simulink model "MPC_LQR"  (R2025b)
settings: Solver=ode4  StartTime=0.0  StopTime=10  FixedStep=0.001  RelTol=1e-3
InitFcn:
  | run("init.m")
settings Model: Creator=aldor  LastModifiedBy=Acer

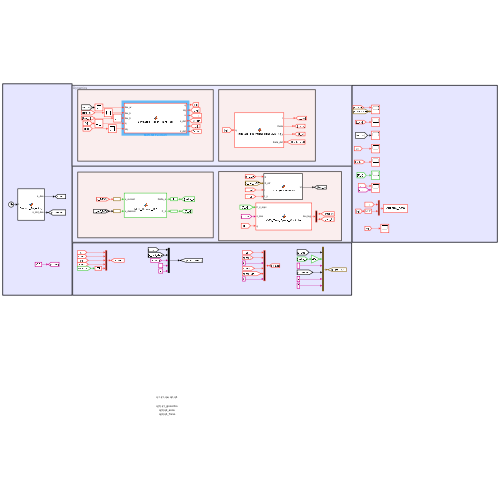
[thumbnail: Simulink's stored preview of the top-level diagram]
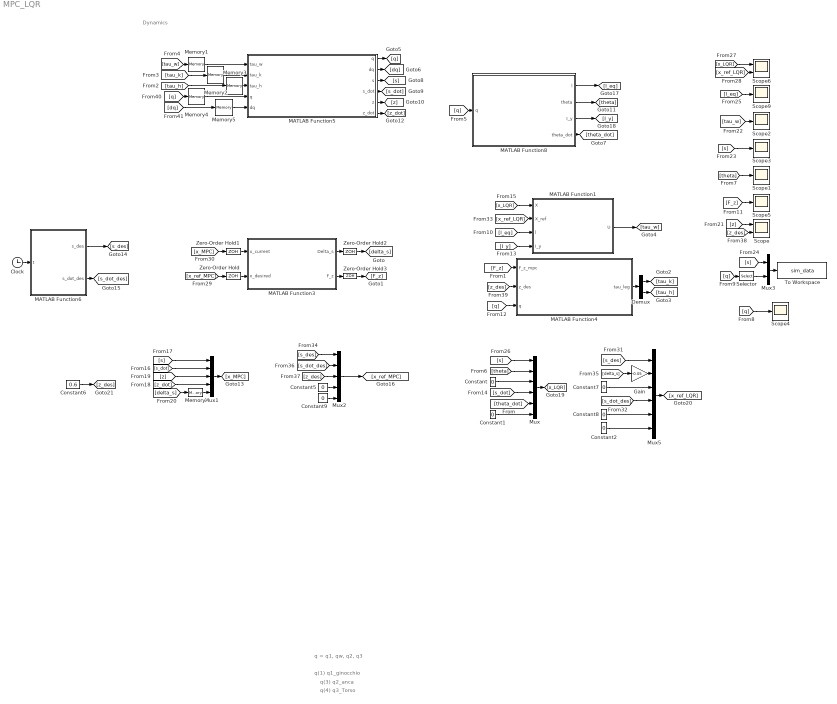
== system MPC_LQR ==
  note: Dynamics
  note: q(3) q2_anca
  note: q(1) q1_ginocchio
  note: q = q1, qw, q2, q3
  note: q(4) q3_Torso
  Clock : Clock
  Constant{,1..2,5,7..9} (7 alike) : Constant  Value=0
  Constant6 : Constant  Value=0.6
  Demux : Demux  Outputs=2
  Gain : Gain  Gain=-0.05
  MATLAB Function1 : MATLAB Function  TreatAsAtomicUnit=on
  MATLAB Function3 : MATLAB Function  TreatAsAtomicUnit=on
  MATLAB Function4 : MATLAB Function  TreatAsAtomicUnit=on
  MATLAB Function5 : MATLAB Function  TreatAsAtomicUnit=on
  MATLAB Function6 : MATLAB Function  TreatAsAtomicUnit=on
  MATLAB Function8 : MATLAB Function  TreatAsAtomicUnit=on
  Memory{,1..5} (6 alike) : Memory
  Mux : Mux  Inputs=6
  Mux1 : Mux  Inputs=5
  Mux2 : Mux  Inputs=5
  Mux3 : Mux  Inputs=[1 3]
  Mux5 : Mux  Inputs=6
  Scope : Scope  NumInputPorts=2
      settings: ActiveDisplayYMinimum=0.1067548531401226  ActiveDisplayYMaximum=0.98813834965109748
  Scope{1..5,9} (6 alike) : Scope
      Scope1 settings: ActiveDisplayYMinimum=-0.026598662061855207  ActiveDisplayYMaximum=0.032394796278817736
      Scope2 settings: ActiveDisplayYMinimum=-998.36065850881471  ActiveDisplayYMaximum=2321.7471304243586  DataLoggingVariableName=ScopeData2
      Scope3 settings: ActiveDisplayYMinimum=-0.15390799680390416  ActiveDisplayYMaximum=1.2448530557444439  DataLoggingVariableName=ScopeData3
      Scope4 settings: ActiveDisplayYMinimum=-1  ActiveDisplayYMaximum=1  DataLoggingVariableName=ScopeData4
      Scope5 settings: ActiveDisplayYMinimum=-792.61159771990333  ActiveDisplayYMaximum=837.79442871292474  DataLoggingVariableName=ScopeData5
      Scope9 settings: ActiveDisplayYMinimum=0.26491553159842146  ActiveDisplayYMaximum=1.1125448908081954  DataLoggingVariableName=ScopeData9
  Scope6 : Scope  NumInputPorts=2
      settings: ActiveDisplayYMinimum=-1  ActiveDisplayYMaximum=1  DataLoggingVariableName=ScopeData6
  Selector : Selector  InputPortWidth=4  IndexOptions=Index vector (dialog)  Indices=[1 3 4]  OutputSizes=1
  To Workspace : ToWorkspace  VariableName=sim_data  SampleTime=-1
  Zero-Order Hold{,1..3} (4 alike) : ZeroOrderHold  SampleTime=1e-2
  wires:
  MATLAB Function4/1(tau_leg) -> Demux/1
  Demux/1 -> [tau_k]
  Demux/2 -> [tau_h]
  MATLAB Function5/1(q) -> [q]
  MATLAB Function5/2(dq) -> [dq]
  MATLAB Function5/5(z) -> [z]
  MATLAB Function5/3(s) -> [s]
  MATLAB Function5/4(s_dot) -> [s_dot]
  [s] -> Mux/1
  Constant/1 -> Mux/3
  [s_dot] -> Mux/4
  Mux/1 -> [x_LQR]
  [x_LQR] -> MATLAB Function1/1(X)
  [x_ref_LQR] -> MATLAB Function1/2(X_ref)
  [s_dot] -> Mux1/2
  [s] -> Mux1/1
  [z] -> Mux1/3
  [z_dot] -> Mux1/4
  [delta_s] -> Memory/1
  Memory/1 -> Mux1/5
  Constant5/1 -> Mux2/4
  Constant9/1 -> Mux2/5
  [tau_w] -> Memory1/1
  Memory1/1 -> MATLAB Function5/1(tau_w)
  Memory2/1 -> MATLAB Function5/2(tau_k)
  [tau_k] -> Memory2/1
  [tau_h] -> Memory3/1
  Memory3/1 -> MATLAB Function5/3(tau_h)
  [z] -> Scope/1
  [z_des] -> Scope/2
  [tau_w] -> Scope2/1
  [s] -> Scope3/1
  Mux3/1 -> To Workspace/1
  [s] -> Mux3/1
  Clock/1 -> MATLAB Function6/1(t)
  MATLAB Function6/1(s_des) -> [s_des]
  [z_des] -> Mux2/3
  [s_des] -> Mux5/1
  [s_dot_des] -> Mux5/4
  Mux5/1 -> [x_ref_LQR]
  [F_z] -> Scope5/1
  [F_z] -> MATLAB Function4/1(F_z_mpc)
  [delta_s] -> Gain/1
  Gain/1 -> Mux5/2
  Mux2/1 -> [x_ref_MPC]
  Zero-Order Hold/1 -> MATLAB Function3/2(x_desired)
  Zero-Order Hold1/1 -> MATLAB Function3/1(x_current)
  Mux1/1 -> [x_MPC]
  Zero-Order Hold2/1 -> [delta_s]
  MATLAB Function3/1(Delta_s) -> Zero-Order Hold2/1
  MATLAB Function3/2(F_z) -> Zero-Order Hold3/1
  Zero-Order Hold3/1 -> [F_z]
  MATLAB Function5/6(z_dot) -> [z_dot]
  [q] -> MATLAB Function4/3(q)
  [q] -> MATLAB Function8/1(q)
  MATLAB Function8/4(theta_dot) -> [theta_dot]
  [theta_dot] -> Mux/5
  Constant1/1 -> Mux/6
  MATLAB Function8/2(theta) -> [theta]
  [theta] -> Mux/2
  [theta] -> Scope1/1
  [q] -> Scope4/1
  [q] -> Selector/1
  Selector/1 -> Mux3/2
  MATLAB Function8/1(l) -> [l_eq]
  [l_eq] -> MATLAB Function1/3(l)
  [l_eq] -> Scope9/1
  MATLAB Function8/3(I_y) -> [I_y]
  [I_y] -> MATLAB Function1/4(I_y)
  [x_LQR] -> Scope6/1
  [x_ref_LQR] -> Scope6/2
  Constant2/1 -> Mux5/6
  Constant8/1 -> Mux5/5
  Constant7/1 -> Mux5/3
  [x_ref_MPC] -> Zero-Order Hold/1
  [x_MPC] -> Zero-Order Hold1/1
  MATLAB Function6/2(s_dot_des) -> [s_dot_des]
  [s_dot_des] -> Mux2/2
  [s_des] -> Mux2/1
  Constant6/1 -> [z_des]
  [z_des] -> MATLAB Function4/2(z_des)
  [q] -> Memory4/1
  [dq] -> Memory5/1
  MATLAB Function1/1(U) -> [tau_w]
  Memory4/1 -> MATLAB Function5/4("q ")
  Memory5/1 -> MATLAB Function5/5("dq ")

== matlab function MPC_LQR/MATLAB Function1 ==
  data: X input; U output; X_ref input; l input; I_y input
function U = TV_LQR_Controller(X, X_ref, l, I_y)
    % X: Stato attuale [s; theta; phi; s_dot; theta_dot; phi_dot] (6x1)
    % X_ref: Stato target desiderato [s_ref; theta_ref; phi_ref; 0; 0; 0] (6x1)
    % l: Lunghezza attuale del pendolo equivalente [m]
    % I_y: Inerzia attuale del corpo superiore [kg*m^2]
    
    % Per usare la funzione lqr() di MATLAB all'interno di Simulink, 
    % dobbiamo dichiararla come estrinseca.
    coder.extrinsic('lqr');
    if l < 0.1
        l = 0.1;
    end
    if I_y < 1e-3
        I_y = 1e-3;
    end
    % 1. Richiamo Parametri Fisici
    m_w = 3.5;       % Massa ruota
    I_w = 0.1;       % Inerzia ruota
    r   = 0.127;     % Raggio ruota
    d   = 0.63;      % Distanza ruote
    m_b = 73.0;      % Massa corpo superiore
    I_z = 3.3;       % Inerzia torso asse z
    g   = 9.81;      % Gravità
    
    % 2. Calcolo dei Coefficienti della Dinamica (Eq. 14)
    % Denominatore comune per a1, a2, b1, b2
    D = 2*I_w*(I_y + m_b*l^2) + (2*l^2*m_b*m_w + I_y*(m_b + 2*m_w)*r^2);
    
    a1 = -(g * l^2 * m_b^2 * r^2) / D;
    a2 =  (g * l * m_b * (2*I_w + (m_b + 2*m_w)*r^2)) / D;
    
    b1 =  (r * (I_y + l*m_b*(l + r))) / D;
    b2 = -(2*I_w + r*(l*m_b + (m_b + 2*m_w)*r)) / D;
    
    % Coefficiente disaccoppiato per lo steering (imbardata)
    b3 =  (d * r) / (2*I_z*r^2 + d^2*(I_w + m_w*r^2));
    
    % 3. Costruzione Matrici di Stato A(l) e Input B(l) (Eq. 12, Eq. 13)
    A = zeros(6, 6);
    A(1, 4) = 1; 
    A(2, 5) = 1; 
    A(3, 6) = 1;
    A(4, 2) = a1;
    A(5, 2) = a2;
    
    B = zeros(6, 2);
    B(4, 1) = b1;  B(4, 2) = b1;
    B(5, 1) = b2;  B(5, 2) = b2;
    B(6, 1) = b3;  B(6, 2) = -b3;
    
    % 4. Definizione Matrici di Peso Q e R (Tuning LQR)
    % Questi valori determinano l'aggressività del controllore. 
    % Possono essere trasformati in input del blocco per un tuning rapido.
    % 4. Definizione Matrici di Peso Q e R (Tuning Soft)
    % Pesi drasticamente ridotti per evitare instabilità con il ritardo discreto
% Aumenta il peso sugli angoli (q1, q2) per evitare che saturino
%X = [s, θ, φ, ṡ, θ̇, φ̇]
    Q = diag([50, 50, 100, 50, 10, 1]);
    R = diag([1, 1]) * 0.5;         % uso coppie piu abbasso piu accelera
    
    % 5. Risoluzione LQR e Calcolo Input
    % Inizializza K per la Code Generation di Simulink
    K = zeros(2, 6); 
    
    % Calcola la matrice dei guadagni ottimali K
    K = lqr(A, B, Q, R);
    
    % Errore di stato (tilde_X)
    X_tilde = X - X_ref;
    
    % Legge di controllo finale (Eq. 16): U = [tau_l; tau_r]
    U = -K * X_tilde; 
end

== matlab function MPC_LQR/MATLAB Function3 ==
  data: x_current input; Delta_s output; x_desired input; F_z output
function [Delta_s, F_z] = MPC_Custom_QP(x_current, x_desired)
    % quadprog non è supportato nativamente per la code generation C
    coder.extrinsic('quadprog');
    coder.extrinsic('optimoptions');

    %% 1. Parametri e Discretizzazione
    m_b = 73.0; 
    g = 9.81;    
    
    h = x_current(3); 
    if h < 0.1
        h = 0.6;
    end
    
    dt = 0.01; 
    N = 40;     
    
    A_c = zeros(5,5);
    A_c(1,2) = 1;
    A_c(3,4) = 1;
    A_c(2,5) = g / h; 
    
    B_c = zeros(5,2);
    B_c(4,2) = 1 / m_b;
    B_c(5,1) = 1;
    
    A_d = eye(5) + A_c * dt;
    B_d = B_c * dt;

    %% 2. Pesi della Funzione di Costo
    %x = [s, ṡ, z, ż, Δs]
    S = diag([1, 1, 500, 50, 1]);
    W = diag([1, 0.01]);

    %% 3. Condensazione (Srotolamento) 
    nx = 5; nu = 2;
    P_x = zeros(nx*N, nx);
    P_u = zeros(nx*N, nu*N);

    A_power = eye(nx);
    for i = 1:N
        A_power = A_power * A_d;
        P_x((i-1)*nx+1 : i*nx, :) = A_power;
        for j = 1:i
            P_u((i-1)*nx+1 : i*nx, (j-1)*nu+1 : j*nu) = (A_d^(i-j)) * B_d;
        end
    end

    S_bar = kron(eye(N), S);
    W_bar = kron(eye(N), W);

    H = 2 * (P_u' * S_bar * P_u + W_bar);
    H = (H + H') / 2; % Garantisce simmetria perfetta
    
    X_ref = repmat(x_desired, N, 1);
    f = 2 * P_u' * S_bar * (P_x * x_current - X_ref);

    %% 4. Vincoli Fisici
    F_min = -1500; % Permette di frenare!
    F_max = 1500;
    
    LB = zeros(nu*N, 1);
    UB = zeros(nu*N, 1);
    
    for i = 1:N
        LB((i-1)*nu+1) = -0.20;   % era -2.0

        UB((i-1)*nu+1) =  0.20;   % era  2.0
 
        
        LB((i-1)*nu+2) = F_min; 
        UB((i-1)*nu+2) = F_max;
    end

    %% 5. Risoluzione QP (CORRETTA)
    % Pre-allocazione per Simulink Coder
    U_opt_calc = zeros(nu*N, 1);
    fval = 0.0;
    exitflag = 0.0;
    
    % Algoritmo robusto di default
    options = optimoptions('quadprog', 'Display', 'off');
    
    % LA CORREZIONE: Aggiunto "fval" per non sballare "exitflag"!
    [U_opt_calc, fval, exitflag] = quadprog(H, f, [], [], [], [], LB, UB, [], options);

    if exitflag > 0
        U_opt = U_opt_calc;
    else
        % Se fallisce davvero, eroga 0 extra, ma il VMC ci terrà in piedi col peso base
        U_opt = zeros(nu*N, 1);
    end

    %% 6. Estrazione Input Ottimo
    Delta_s_dot_opt = U_opt(1);
    F_z = U_opt(2); % FINALMENTE SARA' DIVERSO DA ZERO!

    Delta_s = x_current(5) + Delta_s_dot_opt * dt;
end

== matlab function MPC_LQR/MATLAB Function4 ==
  settings: updateMethod=DISCRETE
  data: tau_leg output size=2; F_z_mpc input size=1; z_des input size=1; q input size=4
function tau_leg  = VMC_Task_Space_Controller(F_z_mpc, z_des, q)

% =========================================================================

% VMC CORRETTO - Ripartizione pulita delle competenze della GAMBA:

%   GINOCCHIO -> altezza z          (canale verticale)

%   ANCA      -> beccheggio torso q3 (stabilizzazione, anello prima mancante)

% Lo spostamento ORIZZONTALE del CoM NON e' piu' gestito qui: e' compito

% della ruota (TV-LQR). Cosi' sparisce il conflitto che destabilizzava l'MPC.

% =========================================================================

    % --- Parametri fisici ---

    l1 = 0.45; l2 = 0.45;

    dt    = 0.001;        % deve coincidere col passo fisso del solutore
 
    % --- Stima derivate via differenza finita (persistenti) ---


 
    % Cinematica utile

    q1_ginocchio=q(1);
    q2_anca=q(3);
    q3_torso=q(4);

        persistent q3_prev z_prev

    if isempty(q3_prev), q3_prev = q3_torso; end

    phi_shank = q1_ginocchio - q2_anca + q3_torso;

    phi_thigh = q3_torso - q2_anca;

    z_actual  = l1*cos(phi_shank) + l2*cos(phi_thigh);
 
    if isempty(z_prev), z_prev = z_actual; end
 
    dq3   = (q3_torso - q3_prev)/dt;   q3_prev = q3_torso;

    z_dot = (z_actual - z_prev)/dt;    z_prev  = z_actual;
 
    % --- CoM: solo per monitoraggio/uscite ---

    coder.extrinsic('calc_com_jacobian');

    J_SC = zeros(1,2); J_ZC = zeros(1,2); SC = 0.0; ZC = 0.0;

    [J_SC, J_ZC, SC, ZC] = calc_com_jacobian(q1_ginocchio, q2_anca, q3_torso);

    SC_out    = SC;

    J_hip_out = J_SC(2);
 
    % --- Compensazione di gravita' dalla dinamica VERA G(q) ---

    % (sostituisce il vecchio Jacobiano del ginocchio "clampato", instabile

    %  a gamba dritta). G non dipende da dq, quindi passo dq = 0.

    coder.extrinsic('calc_dynamics');

    q_full  = [q1_ginocchio; 0; q2_anca; q3_torso];   % ordine [q1;qw;q2;q3]

    M   = zeros(4,4); CdQ = zeros(4,1); G = zeros(4,1);

    [M, CdQ, G] = calc_dynamics(q_full, zeros(4,1));

    tau_k_grav = G(1);   % coppia statica ginocchio

    tau_h_grav = G(3);   % coppia statica anca
 
    % =====================================================================

    % (1) GINOCCHIO  ->  controllo di ALTEZZA

    % =====================================================================

    Kp_z = 4000; Kd_z = 300;               % PD altezza (DA TARARE)

    Jz_knee = -l1*sin(phi_shank);          % dz/dq1

    if abs(Jz_knee) < 0.05                  % vicino a gamba dritta: autorita' ~0

        Jz_knee = 0.05*sign(Jz_knee + 1e-9);

    end

    F_z_cmd = Kp_z*(z_des - z_actual) - Kd_z*z_dot + F_z_mpc;  % forza vert. extra

    tau_k   = tau_k_grav + Jz_knee * F_z_cmd;
 
    % =====================================================================

    % (2) ANCA  ->  stabilizza il BECCHEGGIO del torso  q3 -> 0

    % =====================================================================

    Kp_t = 800; Kd_t = 80;                 % PD torso (DA TARARE)

    % SEGNO: parti con -(Kp*q3 + Kd*dq3). Se in simulazione il torso DIVERGE

    %        invece di raddrizzarsi, INVERTI il segno del termine PD.

    tau_h = tau_h_grav - (Kp_t*q3_torso + Kd_t*dq3);
 
    tau_leg = [tau_k; tau_h];

end

== matlab function MPC_LQR/MATLAB Function5 ==
  data: tau_w input size=2; q output; tau_k input size=1; tau_h input size=1; dq output; s output size=1; s_dot output size=1; z output size=1; z_dot output size=1; q input size=4; dq input size=4
function [q, dq, s, s_dot, z, z_dot] = Simulated_Robot_Plant_Full(tau_w, tau_k, tau_h, q, dq)

    persistent q_static dq_static
    if isempty(q_static)
        q_static  = [0; 0; 0; 0];
        dq_static = [0; 0; 0; 0];
    end

    dt = 0.001;
    limite_gamba = 300;limite_ruota = 50; 
    tau_w_scalar = max(min(tau_w(1)+tau_w(2), limite_ruota), -limite_ruota);
    tau_k_lim    = max(min(tau_k, limite_gamba), -limite_gamba);
    tau_h_lim    = max(min(tau_h, limite_gamba), -limite_gamba);

    tau_vec = [tau_k_lim; tau_w_scalar; tau_h_lim; 0];

    ddq = whole_robot_2D(q, dq, tau_vec);
    dq_static  = dq_static + ddq * dt;
    q_static   = q_static  + dq_static * dt;

    q1_ginocchio = q_static(1);
    q2_anca      = q_static(3);
    q3_torso     = q_static(4); 

    Rw = 0.127;
    s = Rw * q_static(2);
    s_dot    = Rw * dq_static(2);

    l1 = 0.45; l2 = 0.45;
    phi_shank = q1_ginocchio - q2_anca + q3_torso;
    phi_thigh = q3_torso - q2_anca;
    z = l1*cos(phi_shank) + l2*cos(phi_thigh);

    persistent z_prev
    if isempty(z_prev), z_prev = z; end
    z_dot = (z - z_prev)/dt;
    z_prev = z;

    q=q_static;
    dq=dq_static;
end

== matlab function MPC_LQR/MATLAB Function6 ==
  data: t input; s_des output; s_dot_des output
function [s_des, s_dot_des] = Smooth_Trajectory(t)
    % PRE-ALLOCAZIONE PER IL CODER
    s_des = 0.0;
    s_dot_des = 0.0;
    
    % PARAMETRI DELLA TRAIETTORIA
    t_start = 0.0;       % Il robot inizia a muoversi a 2 secondi
    t_end = 5.0;         % Arriva a destinazione a 5 secondi (3 secondi di viaggio)
    s_final = 1.0;       % Destinazione orizzontale (1 metro)
    
    % LOGICA DEL MOVIMENTO
    if t <= t_start
        % Prima di partire, resta fermo
        s_des = 0.0;
        s_dot_des = 0.0;
        
    elseif t >= t_end
        % Arrivato a destinazione, fermati
        s_des = s_final;
        s_dot_des = 0.0;
        
    else
        % FASE DI MOTO: Polinomio Cubico (Minimum Jerk Trajectory)
        % Normalizziamo il tempo tra 0 e 1 per la durata del viaggio
        tau = (t - t_start) / (t_end - t_start);
        
        % Posizione (Profilo a "S" morbida)
        s_des = s_final * (3*tau^2 - 2*tau^3);
        
        % Velocità (Derivata della posizione, forma a campana)
        s_dot_des = s_final * (6*tau - 6*tau^2) / (t_end - t_start);
    end
end

== matlab function MPC_LQR/MATLAB Function8 ==
  data: q input; l output; theta output; I_y output; theta_dot output
function [l, theta, I_y, theta_dot] = calculate_equivalent_pendulum_v3(q)
    persistent theta_prev
    if isempty(theta_prev), theta_prev = 0; end
    dt = 0.001;

    q1_ginocchio = q(1);
    q2_anca = q(3);
    q3_torso = q(4);

    m1=1.2; m2=5.3; m3=60.0;
    l1=0.45; l2=0.45; l3=0.35;

    phi_shank = q1_ginocchio - q2_anca + q3_torso;
    phi_thigh = q3_torso - q2_anca;

    x1 = (l1/2)*sin(phi_shank);              y1 = (l1/2)*cos(phi_shank);
    xk = l1*sin(phi_shank);                  yk = l1*cos(phi_shank);
    x2 = xk + (l2/2)*sin(phi_thigh);         y2 = yk + (l2/2)*cos(phi_thigh);
    xh = xk + l2*sin(phi_thigh);             yh = yk + l2*cos(phi_thigh);
    x3 = xh + (l3/2)*sin(q3_torso);          y3 = yh + (l3/2)*cos(q3_torso);

    m_tot = m1+m2+m3;
    SC = (m1*x1 + m2*x2 + m3*x3) / m_tot;
    ZC = (m1*y1 + m2*y2 + m3*y3) / m_tot;

    l = sqrt(SC^2 + ZC^2);
    if l < 0.1, l = 0.1; end

    theta = atan2(SC, ZC);

    % Unwrap per evitare i falsi picchi di theta_dot
    delta_theta = theta - theta_prev;
    delta_theta = atan2(sin(delta_theta), cos(delta_theta));
    theta_dot = delta_theta / dt;
    theta_prev = theta;

    I_y = (1/3) * m_tot * l^2;
end
